simulink model "lab3"  (R2024a)
settings: Solver=VariableStepAuto  StartTime=0.0  StopTime=1  RelTol=1e-3
libraries: spsRMSLib x3, spsACVoltageSourceLib x1, spsCurrentMeasurementLib x1, spsLinearTransformerLib x1, spsPowerLib x1, spsVoltageMeasurementLib x1, sps_lib x1

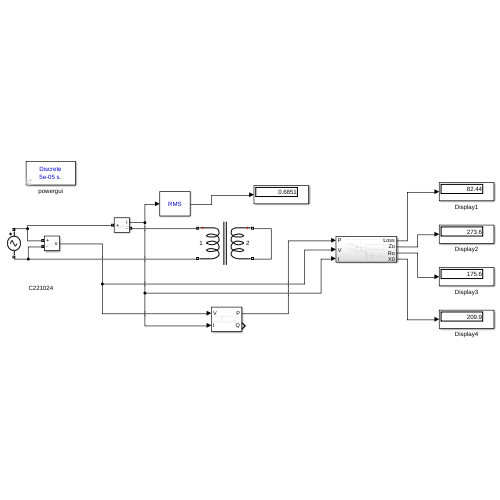
[thumbnail: Simulink's stored preview of the top-level diagram]
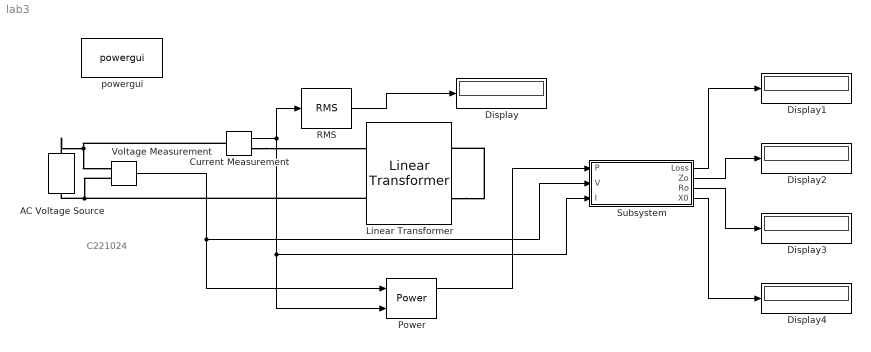
== system lab3 ==
  note: C221024
  AC Voltage Source : spsACVoltageSourceLib/AC Voltage Source  Amplitude=180*sqrt(2)  Phase=0  Frequency=50  SampleTime=0  Measurements=None  BusType=swing  Pref=10e3  Qref=0  Qmin=-inf  Qmax=+inf
  Current Measurement : spsCurrentMeasurementLib/Current Measurement  PhasorSimulation=off  OutputType=Complex  PSBequivalent=0
  Display{,1..4} (5 alike) : Display
  Linear Transformer : spsLinearTransformerLib/Linear Transformer  UNITS=SI  NominalPower=[ 250e6 50 ]  winding1=[5500 20 10e-3]  winding2=[400 5 0.3e-3]  ThreeWindings=off  winding3=[3.15e+05 0.7938 0.084225]  RmLm=[1000 1]  Measurements=None  DataType=on
  Power : spsPowerLib/Power  Freq=60  Vinit=[1, 0]  Iinit=[1, 0]  Ts=0
  RMS : spsRMSLib/RMS  TrueRMS=on  Freq=60  RMSInit=120  Ts=0
  Subsystem : Subsystem
  Voltage Measurement : spsVoltageMeasurementLib/Voltage Measurement  PhasorSimulation=off  OutputType=Complex  PSBequivalent=0
  powergui : sps_lib/powergui  Priority=1  SimulationMode=Discrete  SampleTime=5e-05  frequency=60  Iterations=50  frequencyindice=50  Pbase=100e6  ErrMax=1e-4  UnitsV=kV  UnitsW=MW  buscounter=0  FunctionMessages=off  echomessages=off  EnableUseOfTLC=off  CurrentSourceSwitches=off  DisableSnubberDevices=off  DisableRonSwitches=off  DisableVfSwitches=off  DisplayEquations=off  AutomaticDiscreteSolvers=off  SolverType=Tustin/Backward Euler (TBE)  Interpol=off  ExternalGateDelay=off  methode=off  Ts=100  x0status=blocks  SPID=on  SwTol=0  HookPort=off  NonlinearTolerance=1e-4  nMaxIteration=100  ContinueOnMaxIteration=off  RestoreLinks=warning  ResistiveCurrentMeasurement=off  Frange=[0:2:500]  Ylog=off  Xlog=on  ShowGrid=off  save=off  variable=ZData  structure=0  ZoomFFT=off  StartTime=0.0  cycles=1  DisplayStyle=1  fundamental=60  FreqAxis=off  MaxFrequency=1000  frequencyindicesteady=1  RmsSteady=1  display=off
  wires:
  Current Measurement/1 -> Power/2, Subsystem/3(I), RMS/1
  RMS/1 -> Display/1
  Power/1 -> Subsystem/1(P)
  Subsystem/1(Loss) -> Display1/1
  Subsystem/2(Zo) -> Display2/1
  Subsystem/3(Ro) -> Display3/1
  Subsystem/4(X0) -> Display4/1
  Voltage Measurement/1 -> Subsystem/2(V), Power/1
  connections:
  AC Voltage Source/RConn1 -- Current Measurement/LConn1 -- Voltage Measurement/LConn1
  Linear Transformer/LConn2 -- Voltage Measurement/LConn2 -- AC Voltage Source/LConn1
  Current Measurement/RConn1 -- Linear Transformer/LConn1
  Linear Transformer/RConn2 -- Linear Transformer/RConn1

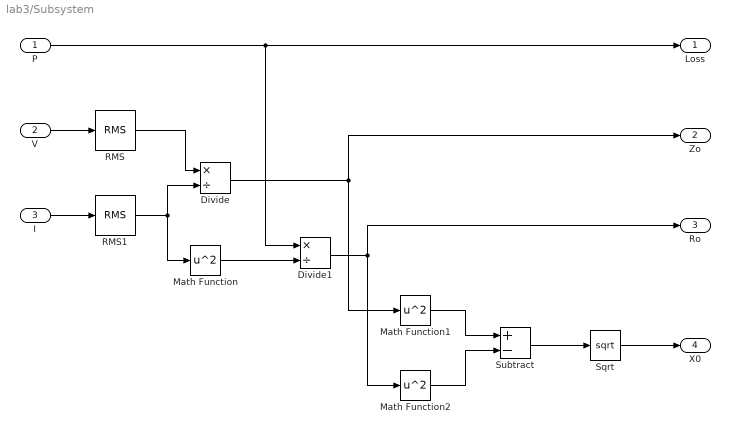
== system lab3/Subsystem ==
  P : Inport
  V : Inport  Port=2
  I : Inport  Port=3
  Divide : Product  Inputs=*/
  Divide1 : Product  Inputs=*/
  Math Function : Math  Operator=square
  Math Function1 : Math  Operator=square
  Math Function2 : Math  Operator=square
  RMS : spsRMSLib/RMS  TrueRMS=on  Freq=60  RMSInit=120  Ts=0
  RMS1 : spsRMSLib/RMS  TrueRMS=on  Freq=60  RMSInit=120  Ts=0
  Sqrt : Sqrt
  Subtract : Sum  Inputs=+-
  Loss : Outport
  Zo : Outport  Port=2
  Ro : Outport  Port=3
  X0 : Outport  Port=4
  wires:
  P/1 -> Divide1/1, Loss/1
  I/1 -> RMS1/1
  V/1 -> RMS/1
  RMS/1 -> Divide/1
  RMS1/1 -> Math Function/1, Divide/2
  Divide/1 -> Math Function1/1, Zo/1
  Math Function/1 -> Divide1/2
  Divide1/1 -> Math Function2/1, Ro/1
  Math Function2/1 -> Subtract/2
  Math Function1/1 -> Subtract/1
  Subtract/1 -> Sqrt/1
  Sqrt/1 -> X0/1
